simulink model "pe_pmsm_drive_code"  (R2018b)
settings: Solver=FixedStepDiscrete  StartTime=0.0  StopTime=0.5  FixedStep=2e-7  MaxStep=2.0E-6  RelTol=1e-6  AbsTol=1e-3  EnableMultiTasking=on
PreLoadFcn:
  | % Control parameters
  | Ts = 2e-6;   % Fundamental sample time
  | fsw = 2e3;   % Switching frequency (Hz)
  | fc = fsw*10; % Control loop frequency (Hz)
  | Tsc = 1/fc;  % Control loop sample time
  | 
  | % PMSM parameters
  | PM = 0.03; % Permanent magnet flux linkage
  | Ld = 2e-4;  % d-axis inductance
  | Lq = 2e-4;  % q-axis inductance
  | L0 = 2e-4;  % 0-axis inductance
  | Rs = 0.013; % Stator resistance
  | N = 6; % Number of pole pairs
  | J = 0.2; % Moment of inertia
  | 
  | % Operating and derived limits
  | Imax = 100;  % Max stator current (peak value)
  | Tmax = 1.5*N*PM*Imax; % Max lectromagnetic torque
  | fnom = 100;  % Nominal frequency (Hz)
  | rpm_nom = 60*fnom/N;      % Nominal rotor speed (rpm)
  | omegam_nom = 2*pi*fnom/N; % Nominal mechanical rotor speed
  | Pmax = omegam_nom*Tmax;     % Maximum power
values from neighbouring files (symbols this model uses):
  faero = 0.5*cd*frontarea*airdens.*speed.^2    [PMSM_code.m]
  speed = linspace(0, 60, 1000)    [PMSM_code.m]
  wheelrad = 0.3    [PMSM_code.m]
undefined symbols (not defined in the file or in its folder): DiscIntNeverNeededParam, gcbh, pe_sli_rtmsupport
libraries: nesl_utility x12, pe_lib x10, fl_lib x8, peTransforms x2, pePmsmCurrentController x1, simulink x1, peVelocityController x1
(part 1 of 2)
CloseFcn:
  | try
  |   clear Imax J L0 Ld Lq N PM Pmax Rs
  |   clear Tmax Ts Tsc fc fnom fsw
  |   clear omegam_nom rpm_nom tout
  | end
Description:
  | Three-Phase PMSM Drive
  | 
  | This example shows a Permanent Magnet Synchronous Machine
  | (PMSM) and inverter sized for use in a typical hybrid vehicle.
  | Here the inverter is connected directly to the vehicle battery, but
  | often there is also a DC-DC converter stage in between. The
  | model can be used to design the PMSM controller, selecting
  | architecture and gains to achieve desired performance. To check
  | the timing of IGBT turn-on and turn-off, the IGBT devices can be
  | directly replaced by more detailed device models from
  | Simscape(TM) Electronics(TM). For complete vehicle modeling, the
  | Simscape Electronics Servomotor block can be used to abstract
  | the PMSM, inverter and controller with an energy-based model.
  | The Gmin resistor provides a very small conductance to ground
  | that improves the numerical properties of the model when using
  | a variable-step solver.
  | 
  | Copyright 2014-2017 The MathWorks, Inc.
settings Model: Creator=The MathWorks, Inc.  LastModifiedBy=Giorgia
settings SolverCC: AutoScaleAbsTol=off  MaxConsecutiveMinStep=2  AlgebraicLoopSolver=LineSearch
settings DataIOCC: LimitDataPoints=on  SaveFormat=Array  ReturnWorkspaceOutputs=on
settings OptimizationCC: DefaultParameterBehavior=Inlined  UseDivisionForNetSlopeComputation=on  UseFloatMulNetSlope=on  InlineInvariantSignals=on  PassReuseOutputArgsAs=Individual arguments  ZeroExternalMemoryAtStartup=off  ZeroInternalMemoryAtStartup=off  NoFixptDivByZeroProtection=on  EfficientFloat2IntCast=on  LifeSpan=1  OptimizeBlockOrder=speed  DifferentSizesBufferReuse=on
settings DebuggingCC: UnderspecifiedInitializationDetection=Classic  MergeDetectMultiDrivingBlocksExec=none  MaxConsecutiveZCsMsg=none  ParameterTunabilityLossMsg=error  AllowSymbolicDim=off  LibraryContextMissingDiagnostic=none  SFUnexpectedBacktrackingDiag=warning  SFNoUnconditionalDefaultTransitionDiag=warning  SFExecutionAtInitializationDiag=none
settings HardwareCC: ProdBitPerPointer=32  ProdBitPerSizeT=32  ProdBitPerPtrDiffT=32  ProdLargestAtomicInteger=Long  ProdLargestAtomicFloat=Double  ProdWordSize=32  ProdLongLongMode=on  ProdHWDeviceType=ARM Compatible->ARM Cortex
settings ModelReferenceCC: PropagateSignalLabelsOutOfModel=off
settings SFSimCC: SimUseLocalCustomCode=off  MATLABDynamicMemAlloc=off
settings RTWCC: SystemTargetFile=autosar.tlc  GenCodeOnly=on  TemplateMakefile=ert_default_tmf  Description=AUTOSAR  GenerateReport=on  RTWUseLocalCustomCode=off  IncludeHyperlinkInReport=on  LaunchReport=on  GenerateTraceInfo=on  GenerateTraceReport=on  GenerateTraceReportSl=on  GenerateTraceReportSf=on  GenerateTraceReportEml=on  GenerateCodeMetricsReport=on
settings CodeAppCC: ForceParamTrailComments=on  IgnoreCustomStorageClasses=off  OperatorAnnotations=on  SimulinkDataObjDesc=on  SFDataObjDesc=on  CustomSymbolStrGlobalVar=rt$N$M  CustomSymbolStrType=$N$M  CustomSymbolStrFcn=$N$M$F  CustomSymbolStrMacro=$N$M  InsertBlockDesc=on
settings STFCustomTargetCC: MultiwordLength=256  ParMdlRefBuildCompliant=on  CompOptLevelCompliant=on  IncludeMdlTerminateFcn=off  CombineOutputUpdateFcns=on  CombineSignalStateStructs=on  SuppressErrorStatus=on  ERTCustomFileBanners=on  SupportNonFinite=off  SupportComplex=off  SupportContinuousTime=off  SupportNonInlinedSFcns=off  RemoveResetFunc=on  MATLABClassNameForMDSCustomization=Simulink.SoftwareTarget.ERTCustomization  AutosarCompliant=on  UseToolchainInfoCompliant=on  LookupTableObjectStructAxisOrder=2,1,3,4,...  LUTObjectStructOrderEvenSpacing=Size,Table,Breakpoints  SystemTargetFile=autosar.tlc
settings ERTTargetCC: ConcurrentExecutionCompliant=off  IncludeMdlTerminateFcn=off  CombineSignalStateStructs=on  SuppressErrorStatus=on  SupportNonFinite=off  SupportComplex=off  ModelStepFunctionPrototypeControlCompliant=off  CPPClassGenCompliant=off  AutosarCompliant=on  LookupTableObjectStructAxisOrder=2,1,3,4,...  LUTObjectStructOrderEvenSpacing=Size,Table,Breakpoints  InlinedParameterPlacement=NonHierarchical  ERTCustomFileTemplate=example_file_process.tlc
settings ConfigComp: CovMetricSettings=dw  CovHtmlReporting=on  CovSaveCumulativeToWorkspaceVar=on  CovSaveSingleToWorkspaceVar=on  CovShowResultsExplorer=off  CovExternalEMLEnable=off  CovSFcnEnable=off

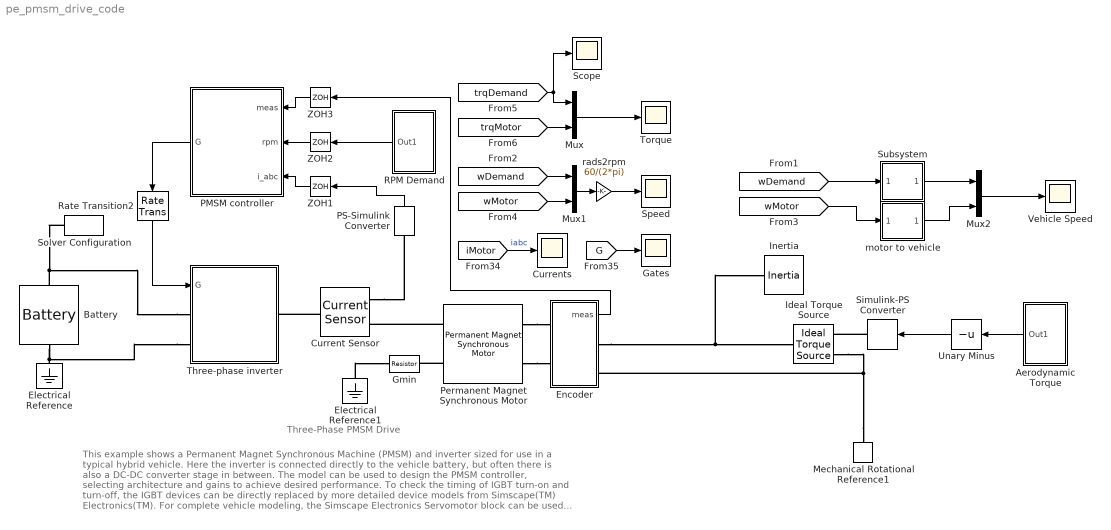
== system pe_pmsm_drive_code ==
  note: This example shows a Permanent Magnet Synchronous Machine (PMSM) and inverter sized for use in a typical hybrid vehicle.
      | Here the inverter is connected directly to the vehicle battery, but often there is also a DC-DC converter stage in between. The
      | model can be used to design the PMSM controller, selecting architecture and gains to achieve desired performance. To check
      | the timing of IGBT turn-on and turn-off, the IGBT devices can be directly replaced by more detailed device models from
      | Simscape(TM) Electronics(TM). For complete vehicle modeling, the Simscape Electronics Servomotor block can be used to
      | abstract the PMSM, inverter and controller with an energy-based model. The Gmin resistor provides a very small conductance
      | to ground that improves the numerical properties of the model when using a variable-step solver.
  note: Three-Phase PMSM Drive
  Aerodynamic Torque : Subsystem
  Battery : pe_lib/Sources/Battery  Vnom=110 V  R1=0.001 Ohm  prm_AH=1  AH=14000 hr*A  V1=470 V  AH1=5000 hr*A  prm_R2=1  R2=inf Ohm  prm_dyn=1  Rp1=0.005 Ohm  tau1=30 s  Rp2=0.005 Ohm  tau2=30 s  Rp3=0.005 Ohm  tau3=30 s  Rp4=0.005 Ohm  tau4=30 s  Rp5=0.005 Ohm  tau5=30 s  prm_fade=1  N_fade=100  AH_fade=45 hr*A  R1_fade=2.02 Ohm  V1_fade=10.35 V  i_specify=off  i_priority=None  i=0 A  i_nominal_specify=off  i_nominal_unit=A  i_nominal_value=1  v_specify=off  v_priority=None  v=0 V  v_nominal_specify=off  v_nominal_unit=V  v_nominal_value=1  charge_specify=on  charge_priority=High  charge=7000 hr*A  charge_nominal_specify=off  charge_nominal_unit=hr*A  charge_nominal_value=1  num_cycles_specify=off  num_cycles_priority=High  num_cycles=0  num_cycles_nominal_specify=off  num_cycles_nominal_unit=1  num_cycles_nominal_value=1  thermal_mass=30000 J/K  Tmeas=298.15 K  Vnom_T2=12 V  R1_T2=2.2 Ohm  V1_T2=11.4 V  R2_T2=2200 Ohm  Rp1_T2=0.005 Ohm  tau1_T2=30 s  Rp2_T2=0.005 Ohm  tau2_T2=30 s  Rp3_T2=0.005 Ohm  tau3_T2=30 s  Rp4_T2=0.005 Ohm  tau4_T2=30 s  Rp5_T2=0.005 Ohm  tau5_T2=30 s  Tmeas2=273.15 K  temperature_specify=off  temperature_priority=High  temperature=298.15 K  temperature_nominal_specify=off  temperature_nominal_unit=K  temperature_nominal_value=1
      settings: SourceProductName=Simscape Electrical  SourceProductBaseCode=PS
  Current Sensor : pe_lib/Sensors/Current Sensor
      settings: SourceProductName=Simscape Electrical  SourceProductBaseCode=PS
  Currents : Scope
  Electrical Reference : fl_lib/Electrical/Electrical Elements/Electrical Reference
      settings: SourceProductName=Foundation Library
  Electrical Reference1 : fl_lib/Electrical/Electrical Elements/Electrical Reference
      settings: SourceProductName=Foundation Library
  Encoder : Subsystem
  Gates : Scope
  Gmin : fl_lib/Electrical/Electrical Elements/Resistor  R=1e9 Ohm  i_specify=off  i_priority=High  i=0 A  i_nominal_specify=off  i_nominal_unit=A  i_nominal_value=1  v_specify=off  v_priority=High  v=0 V  v_nominal_specify=off  v_nominal_unit=V  v_nominal_value=1
      settings: SourceProductName=Foundation Library
  Ideal Torque Source : fl_lib/Mechanical/Mechanical Sources/Ideal Torque Source
  Inertia : fl_lib/Mechanical/Rotational Elements/Inertia  inertia=0.01 kg*m^2  w_specify=off  w_priority=High  w=0 rad/s  w_nominal_specify=off  w_nominal_unit=rad/s  w_nominal_value=1  t_specify=off  t_priority=None  t=0 N*m  t_nominal_specify=off  t_nominal_unit=N*m  t_nominal_value=1
  Mechanical Rotational Reference1 : fl_lib/Mechanical/Rotational Elements/Mechanical Rotational Reference
      settings: SourceProductName=Foundation Library
  Mux : Mux  Inputs=2
  Mux1 : Mux  Inputs=2
  Mux2 : Mux  Inputs=2
  PMSM controller : Subsystem
  PS-Simulink Converter : nesl_utility/PS-Simulink Converter  PhysicalDomain=network_engine_domain  SubClassName=ps_output  LeftPortType=input  RightPortType=output  PseudoPeriodic=off  Frequencies=[]  Unit=A  AffineConversion=off
  Permanent Magnet Synchronous Motor : pe_lib/Machines/Permanent Magnet Rotor/Permanent Magnet Synchronous Motor  nPolePairs=N  pmflux_param=1  pm_flux_linkage=PM Wb  torque_constant=0.18 N*m/A  back_emf_constant=0.18 V/(rad/s)  stator_param=1  Ld=Ld H  Lq=Lq H  L0=L0 H  Ls=0.0002 H  Lm=0.00002 H  Ms=0.00002 H  Rs=Rs Ohm  zero_sequence=pe.enum.park.zerosequence.include  J=0 kg*m^2  lam=0 N*m/(rad/s)  axes_param=1  i_d_specify=off  i_d_priority=None  i_d=0 A  i_d_nominal_specify=off  i_d_nominal_unit=A  i_d_nominal_value=1  i_q_specify=off  i_q_priority=None  i_q=0 A  i_q_nominal_specify=off  i_q_nominal_unit=A  i_q_nominal_value=1  torque_specify=off  torque_priority=None  torque=0 N*m  torque_nominal_specify=off  torque_nominal_unit=N*m  torque_nominal_value=1  angular_velocity_specify=on  angular_velocity_priority=None  angular_velocity=0 rpm  angular_velocity_nominal_specify=off  angular_velocity_nominal_unit=rpm  angular_velocity_nominal_value=1  angular_position_specify=on  angular_position_priority=High  angular_position=0 rad  angular_position_nominal_specify=off  angular_position_nominal_unit=deg  angular_position_nominal_value=1
      settings: SourceProductName=Simscape Electrical  SourceProductBaseCode=PS
  RPM Demand : Subsystem
  Rate Transition2 : RateTransition  Deterministic=off  OutPortSampleTime=Ts
  Scope : Scope
  Simulink-PS Converter : nesl_utility/Simulink-PS Converter  PhysicalDomain=network_engine_domain  SubClassName=ps_input  LeftPortType=input  RightPortType=output  PseudoPeriodic=off  Frequencies=[]  NoiseDistribution=none  NoiseParameters=[]  Unit=1  AffineConversion=off  FilteringAndDerivatives=provide  SimscapeFilterOrder=1  InputFilterTimeConstant=0.001  UdotUserProvided=0
  Solver Configuration : nesl_utility/Solver Configuration  PhysicalDomain=network_engine_domain  SubClassName=solver  LeftPortType=input  RightPortType=generic  Tones=[]  Harmonics=[]  SimulateNoise=off  Profile=off  UseLocalSampling=off  EnableSwitchedLinearOptims=on  FrequencyDomain=off  UseCCode=off  RelTol=0.001  AbsTol=1e-06  MinStep=1e-09  ToWorkspace=off  RevertToSquareIcSolve=off  NumHomotopyIterations=100  PhasorMode=off  PhasorModeNumHarmonics=1  DoDC=off  ResidualTolerance=1e-9  UseLocalSolver=on  LocalSolverChoice=NE_BACKWARD_EULER_ADVANCER  LocalSolverSampleTime=Ts  DoFixedCost=on  MaxNonlinIter=4  MaxModeIter=2  LinearAlgebra=Sparse  EquationFormulation=NE_TIME_EF  DelaysMemoryBudget=1024  AutomaticFiltering=on  FilteringTimeConstant=0.001  PartitionStorageMethod=AS_NEEDED  PartitionMemoryBudget=1024
  Speed : Scope
  Subsystem : Subsystem
  Three-phase inverter : Subsystem
  Torque : Scope
  Unary Minus : UnaryMinus
  "Vehicle Speed " : Scope
  ZOH1 : ZeroOrderHold  SampleTime=Tsc
  ZOH2 : ZeroOrderHold  SampleTime=Tsc
  ZOH3 : ZeroOrderHold  SampleTime=Tsc
  "motor to vehicle " : Subsystem
  rads2rpm : Gain  Gain=60/(2*pi)
  wires:
  PS-Simulink Converter/1 -> ZOH1/1
  Mux1/1 -> rads2rpm/1
  [iMotor] -> Currents/1  "iabc"
  [G] -> Gates/1
  [wDemand] -> Mux1/1
  Mux/1 -> Torque/1
  [trqMotor] -> Mux/2
  [trqDemand] -> Scope/1, Mux/1
  Encoder/1(meas) -> ZOH3/1
  ZOH3/1 -> PMSM controller/1(meas)
  ZOH2/1 -> PMSM controller/2(rpm)
  ZOH1/1 -> PMSM controller/3(i_abc)
  Rate Transition2/1 -> Three-phase inverter/1(G)
  [wMotor] -> Mux1/2
  rads2rpm/1 -> Speed/1
  PMSM controller/1(G) -> Rate Transition2/1
  Aerodynamic Torque/1(Out1) -> Unary Minus/1
  Unary Minus/1 -> Simulink-PS Converter/1
  Mux2/1 -> "Vehicle Speed "/1
  [wDemand] -> Subsystem/1(In1)
  Subsystem/1(Out1) -> Mux2/1
  [wMotor] -> "motor to vehicle "/1(In1)
  "motor to vehicle "/1(Out1) -> Mux2/2
  RPM Demand/1(Out1) -> ZOH2/1
  connections:
  Three-phase inverter/LConn1 -- Solver Configuration/RConn1 -- Battery/LConn1
  Permanent Magnet Synchronous Motor/RConn1 -- Encoder/LConn1
  Permanent Magnet Synchronous Motor/RConn2 -- Encoder/LConn2
  Current Sensor/LConn1 -- Three-phase inverter/RConn1
  Three-phase inverter/LConn2 -- Electrical Reference/LConn1 -- Battery/RConn1
  Permanent Magnet Synchronous Motor/LConn1 -- Current Sensor/RConn2
  Current Sensor/RConn1 -- PS-Simulink Converter/LConn1
  Permanent Magnet Synchronous Motor/LConn2 -- Gmin/RConn1
  Electrical Reference1/LConn1 -- Gmin/LConn1
  Encoder/RConn1 -- Ideal Torque Source/LConn1 -- Inertia/LConn1
  Mechanical Rotational Reference1/LConn1 -- Ideal Torque Source/RConn2 -- Encoder/RConn2
  Simulink-PS Converter/RConn1 -- Ideal Torque Source/RConn1

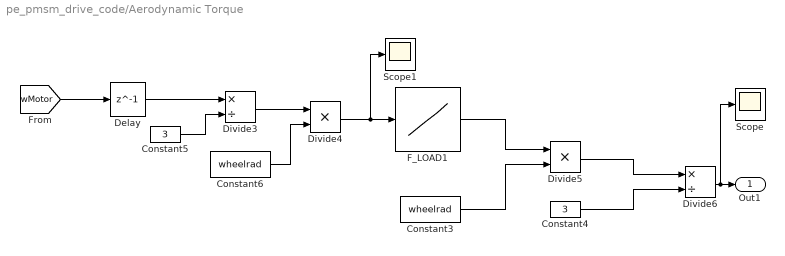
== system pe_pmsm_drive_code/Aerodynamic Torque ==
  Constant3 : Constant  Value=wheelrad
  Constant4 : Constant  Value=3
  Constant5 : Constant  Value=3
  Constant6 : Constant  Value=wheelrad
  Delay : Delay  DelayLength=1  InitialCondition=0
  Divide3 : Product  Inputs=*/
  Divide4 : Product  Inputs=**
  Divide5 : Product  Inputs=**
  Divide6 : Product  Inputs=*/
  F_LOAD1 : Lookup_n-D  NumberOfTableDimensions=1  BreakpointsForDimension1=speed  Table=faero  ExtrapMethod=Clip  RemoveProtectionInput=on  UseLastTableValue=on  InternalRulePriority=Speed  RndMeth=Simplest  InputSameDT=on
  Scope : Scope
  Scope1 : Scope
  Out1 : Outport
  wires:
  F_LOAD1/1 -> Divide5/1
  Constant3/1 -> Divide5/2
  Divide5/1 -> Divide6/1
  Constant4/1 -> Divide6/2
  Divide6/1 -> Scope/1, Out1/1
  Constant5/1 -> Divide3/2
  Delay/1 -> Divide3/1
  Divide3/1 -> Divide4/1
  Constant6/1 -> Divide4/2
  Divide4/1 -> Scope1/1, F_LOAD1/1
  [wMotor] -> Delay/1

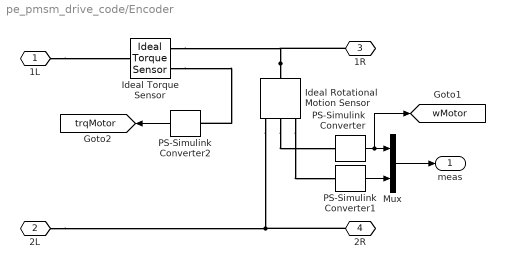
== system pe_pmsm_drive_code/Encoder ==
  Ideal Rotational Motion Sensor : fl_lib/Mechanical/Mechanical Sensors/Ideal Rotational Motion Sensor  offset=0 deg
      settings: SourceProductName=Foundation Library
  Ideal Torque Sensor : fl_lib/Mechanical/Mechanical Sensors/Ideal Torque Sensor
      settings: SourceProductName=Foundation Library
  Mux : Mux  Inputs=2
  PS-Simulink Converter : nesl_utility/PS-Simulink Converter  PhysicalDomain=network_engine_domain  SubClassName=ps_output  LeftPortType=input  RightPortType=output  PseudoPeriodic=off  Frequencies=[]  Unit=rad/s  AffineConversion=off
  PS-Simulink Converter1 : nesl_utility/PS-Simulink Converter  PhysicalDomain=network_engine_domain  SubClassName=ps_output  LeftPortType=input  RightPortType=output  PseudoPeriodic=off  Frequencies=[]  Unit=rad  AffineConversion=off
  PS-Simulink Converter2 : nesl_utility/PS-Simulink Converter  PhysicalDomain=network_engine_domain  SubClassName=ps_output  LeftPortType=input  RightPortType=output  PseudoPeriodic=off  Frequencies=[]  Unit=N*m  AffineConversion=off
  1L : PMIOPort  Side=Left
  2L : PMIOPort  Port=2  Side=Left
  1R : PMIOPort  Port=3  Side=Right
  2R : PMIOPort  Port=4  Side=Right
  meas : Outport
  tag scope: trqMotor=global, wMotor=global
  wires:
  PS-Simulink Converter2/1 -> [trqMotor]
  Mux/1 -> meas/1
  PS-Simulink Converter1/1 -> Mux/2
  PS-Simulink Converter/1 -> [wMotor], Mux/1
  connections:
  Ideal Torque Sensor/RConn2 -- PS-Simulink Converter2/LConn1
  1L/RConn1 -- Ideal Torque Sensor/LConn1
  2R/RConn1 -- 2L/RConn1 -- Ideal Rotational Motion Sensor/RConn1
  Ideal Rotational Motion Sensor/LConn1 -- 1R/RConn1 -- Ideal Torque Sensor/RConn1
  Ideal Rotational Motion Sensor/RConn2 -- PS-Simulink Converter/LConn1
  Ideal Rotational Motion Sensor/RConn3 -- PS-Simulink Converter1/LConn1

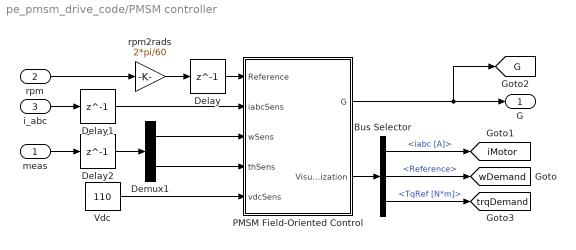
== system pe_pmsm_drive_code/PMSM controller ==
  meas : Inport
  rpm : Inport  Port=2
  i_abc : Inport  Port=3
  Bus Selector : BusSelector  OutputSignals=iabc [A],Reference,TqRef [N*m]
  Delay : Delay  DelayLength=1  InitialCondition=0
  Delay1 : Delay  DelayLength=1  InitialCondition=0
  Delay2 : Delay  DelayLength=1  InitialCondition=0
  Demux1 : Demux  Outputs=2
  PMSM Field-Oriented Control : Subsystem  AncestorBlock=pePmsmFieldOrientedControl/PMSM Field-Oriented Control  LoadFcn=pe_sli_rtmsupport( 'loadfcn', gcbh );  mask(PMSM Field-Oriented Control){CtrlMode=Velocity control, Vnom=110, Pmax=Pmax, Tmax=Tmax*1.5, p=N, Vdc_on=10, Ts=Ts, Tsc=Tsc, CtrlType=PI control, Kp_w=0.8, Ki_w=20, Kv_w=1, Kaw_w=1000, RefType=Zero d-axis control, rpmVec=[0, 3000], TqVec=[-100, 0, 100], VdcVec=[300, 350], idMatrix=zeros(2,3,2), iqMatrix=zeros(2,3,2), psim=PM, Ld=0.00024, Lq=0.00029, Rs=0.01, AxisAlignment=Q-axis, Kp_id=0.1, Ki_id=10, Kaw_id=1000, Kp_iq=0.1, Ki_iq=10, Kaw_iq=1000, AxisPrio=Q-axis, ActZC=off, ActFF=on, ParamTypeFF=Constant parameters, LdFF=Ld, LqFF=Lq, psimFF=PM, idVect=[-200, 0, 200], iqVect=[-200, 0, 200], LdMatrix=0.0002 * ones(3, 3), LqMatrix=0.0002 * ones(3, 3), psimMatrix=0.04 * ones(3, 3), CPWMMode=SPWM: sinusoidal PWM, SamplingMode=Natural, fsw=fsw}
      mask prompts: CtrlMode "Control mode:"; Vnom "Nominal dc-link voltage (V):"; Pmax "Maximum power (W):"; Tmax "Maximum torque (N*m):"; p "Number of rotor pole pairs:"; Vdc_on "Inverter dc-link voltage threshold (V):"; Ts "Fundamental sample time (s):"; Tsc "Control sample time (s):"; CtrlType "Control type:"; Kp_w "Controller proportional gain:"; Ki_w "Controller integral gain:"; Kv_w "P controller proportional gain:"; Kaw_w "Integral anti-windup gain:"; RefType "Current references:"; rpmVec "Mechanical speed vector, wMechanical (rpm):"; TqVec "Torque reference vector, TqRef (N*m):"; VdcVec "DC-link voltage vector, Vdc (V)"; idMatrix "D-axis current reference matrix, id(wMechanical,TqRef,Vdc), (A):"; iqMatrix "Q-axis current reference matrix, iq(wMechanical,TqRef,Vdc), (A):"; psim "Permanent magnet flux linkage (Wb):"; Ld "D-axis inductance (H):"; Lq "Q-axis inductance (H):"; Rs "Stator resistance (Ohm):"; AxisAlignment "Phase-a axis alignment:"; Kp_id "D-axis current proportional gain:"; Ki_id "D-axis current integral gain:"; Kaw_id "D-axis current anti-windup gain:"; Kp_iq "Q-axis current proportional gain:"; Ki_iq "Q-axis current integral gain:"; Kaw_iq "Q-axis current anti-windup gain:"; AxisPrio "Axis prioritization:"; ActZC "Enable zero cancellation"; ActFF "Enable pre-control voltage"; ParamTypeFF "Machine parameters:"; LdFF "D-axis inductance for feed-forward pre-control (H):"; LqFF "Q-axis inductance for feed-forward pre-control (H):"; psimFF "Permanent magnet flux linkage for feed-forward pre-control (Wb):"; idVect "D-axis current vector, id (A):"; iqVect "Q-axis current vector, iq (A):"; LdMatrix "Ld matrix, Ld(id,iq), (H):"; LqMatrix "Lq matrix, Lq(id,iq), (H):"; psimMatrix "Permanent magnet flux linkage matrix, PM(id,iq), (Wb):"; CPWMMode "PWM method:"; SamplingMode "Sampling mode:"; fsw "Switching frequency (Hz):"
      mask help: This block implements a PMSM field-oriented control structure.
      mask init:
      | if ParamTypeFF == 1
      |     idVect = [-200, 200];
      |     iqVect = [-200, 200];
      |     LdMatrix = LdFF*ones(2, 2);
      |     LqMatrix = LqFF*ones(2, 2);
      |     psimMatrix = psimFF*ones(2, 2);
      | end
      settings: CopyFcn=pe_sli_rtmsupport( 'copyfcn', gcbh );  DeleteFcn=pe_sli_rtmsupport( 'deletefcn', gcbh );  ModelCloseFcn=pe_sli_rtmsupport( 'modelclosefcn', gcbh );  PostSaveFcn=pe_sli_rtmsupport( 'postsavefcn', gcbh );  PreCopyFcn=pe_sli_rtmsupport( 'precopyfcn', gcbh );  OpenFcn=pe_sli_rtmsupport( 'openfcn', gcbh );  CloseFcn=pe_sli_rtmsupport( 'closefcn', gcbh );  PreDeleteFcn=pe_sli_rtmsupport( 'predeletefcn', gcbh );
      mask Help: web(nesl_help(gcbh))
      mask TypeOptions CtrlMode: Velocity control | Torque control
      mask Callback CtrlMode: pe.mask.callbackPopupPmsmFoc(gcb);
      mask TypeOptions Vnom:
      | Outer loop control/PMSM Current Reference
      | Generator/Vnom
      mask TypeOptions Pmax:
      | Outer loop control/PMSM Current Reference
      | Generator/Pmax
      mask TypeOptions Tmax:
      | Outer loop control/PMSM Current Reference
      | Generator/Tmax
      mask TypeOptions CtrlType: Outer loop control/Velocity Controller/CtrlType
      mask Callback CtrlType: pe.mask.callbackPopupPmsmFoc(gcb);
      mask TypeOptions Kp_w: Outer loop control/Velocity Controller/Kp_w
      mask TypeOptions Ki_w: Outer loop control/Velocity Controller/Ki_w
      mask TypeOptions Kv_w: Outer loop control/Velocity Controller/Kv_w
      mask TypeOptions Kaw_w: Outer loop control/Velocity Controller/Kaw_w
      mask TypeOptions RefType:
      | Outer loop control/PMSM Current Reference
      | Generator/RefType
      mask Callback RefType: pe.mask.callbackPopupPmsmFoc(gcb);
      mask TypeOptions rpmVec:
      | Outer loop control/PMSM Current Reference
      | Generator/rpmVec
      mask TypeOptions TqVec:
      | Outer loop control/PMSM Current Reference
      | Generator/TqVec
      mask TypeOptions VdcVec:
      | Outer loop control/PMSM Current Reference
      | Generator/VdcVec
      mask TypeOptions idMatrix:
      | Outer loop control/PMSM Current Reference
      | Generator/idMatrix
      mask TypeOptions iqMatrix:
      | Outer loop control/PMSM Current Reference
      | Generator/iqMatrix
      mask TypeOptions psim:
      | Outer loop control/PMSM Current Reference
      | Generator/psim
      mask TypeOptions Ld:
      | Outer loop control/PMSM Current Reference
      | Generator/Ld
      mask TypeOptions Lq:
      | Outer loop control/PMSM Current Reference
      | Generator/Lq
      mask TypeOptions Rs:
      | Outer loop control/PMSM Current Reference
      | Generator/Rs
      mask TypeOptions AxisAlignment: Inner loop control/Park Transform/AxisAlignment
      mask TypeOptions Kp_id:
      | Inner loop control/PMSM Current Controller
      | with Pre-Control/Kp_id
      mask TypeOptions Ki_id:
      | Inner loop control/PMSM Current Controller
      | with Pre-Control/Ki_id
      mask TypeOptions Kaw_id:
      | Inner loop control/PMSM Current Controller
      | with Pre-Control/Kaw_id
      mask TypeOptions Kp_iq:
      | Inner loop control/PMSM Current Controller
      | with Pre-Control/Kp_iq
      mask TypeOptions Ki_iq:
      | Inner loop control/PMSM Current Controller
      | with Pre-Control/Ki_iq
      mask TypeOptions Kaw_iq:
      | Inner loop control/PMSM Current Controller
      | with Pre-Control/Kaw_iq
      mask TypeOptions AxisPrio:
      | Inner loop control/PMSM Current Controller
      | with Pre-Control/AxisPrio
      mask TypeOptions ActZC:
      | Inner loop control/PMSM Current Controller
      | with Pre-Control/ActZC
      mask TypeOptions ActFF:
      | Inner loop control/PMSM Current Controller
      | with Pre-Control/ActFF
      mask Callback ActFF: pe.mask.callbackPopupPmsmFoc(gcb);
      mask TypeOptions ParamTypeFF: Constant parameters | Lookup table based parameters
      mask Callback ParamTypeFF: pe.mask.callbackPopupPmsmFoc(gcb);
      mask TypeOptions idVect:
      | Inner loop control/PMSM Current Controller
      | with Pre-Control/idVect
      mask TypeOptions iqVect:
      | Inner loop control/PMSM Current Controller
      | with Pre-Control/iqVect
      mask TypeOptions LdMatrix:
      | Inner loop control/PMSM Current Controller
      | with Pre-Control/LdMatrix
      mask TypeOptions LqMatrix:
      | Inner loop control/PMSM Current Controller
      | with Pre-Control/LqMatrix
      mask TypeOptions psimMatrix:
      | Inner loop control/PMSM Current Controller
      | with Pre-Control/psimMatrix
      mask TypeOptions CPWMMode:
      | PWM/PWM Generator
      | (Three-phase, Two-level)/CPWMMode
      mask TypeOptions SamplingMode:
      | PWM/PWM Generator
      | (Three-phase, Two-level)/SamplingMode
      mask DialogControl Container4 Prompt: General
      mask DialogControl Container7 Prompt: Outer Loop
      mask DialogControl Container8 Prompt: Inner Loop
      mask DialogControl Container9 Prompt: PWM
  Vdc : Constant  Value=110  SampleTime=Tsc
  rpm2rads : Gain  Gain=2*pi/60
  G : Outport
  tag scope: G=global, iMotor=global, trqDemand=global, wDemand=global
  wires:
  PMSM Field-Oriented Control/1(G) -> G/1, [G]
  Vdc/1 -> PMSM Field-Oriented Control/5(vdcSens)
  PMSM Field-Oriented Control/2(Visualization) -> Bus Selector/1
  i_abc/1 -> Delay1/1
  meas/1 -> Delay2/1
  Demux1/2 -> PMSM Field-Oriented Control/4(thSens)
  Bus Selector/1 -> [iMotor]  "<iabc [A]>"
  Bus Selector/2 -> [wDemand]  "<Reference>"
  Bus Selector/3 -> [trqDemand]  "<TqRef [N*m]>"
  rpm/1 -> rpm2rads/1
  rpm2rads/1 -> Delay/1
  Demux1/1 -> PMSM Field-Oriented Control/3(wSens)
  Delay/1 -> PMSM Field-Oriented Control/1(Reference)
  Delay1/1 -> PMSM Field-Oriented Control/2(iabcSens)
  Delay2/1 -> Demux1/1

== system pe_pmsm_drive_code/RPM Demand ==
  Constant3 : Constant  Value=wheelrad
  Constant4 : Constant  Value=3
  Divide5 : Product  Inputs=*/
  Divide6 : Product  Inputs=**
  Gain2 : Gain  Gain=30/pi
  Scope : Scope
  Scope1 : Scope
  Step : Step  Time=0.1  After=15  SampleTime=Tsc
  Out1 : Outport
  wires:
  Step/1 -> Scope/1, Divide5/1
  Constant4/1 -> Divide6/2
  Divide6/1 -> Gain2/1
  Divide5/1 -> Divide6/1
  Constant3/1 -> Divide5/2
  Gain2/1 -> Scope1/1, Out1/1

== system pe_pmsm_drive_code/Subsystem ==
  In1 : Inport
  Constant5 : Constant  Value=3
  Constant6 : Constant  Value=wheelrad
  Divide3 : Product  Inputs=*/
  Divide4 : Product  Inputs=**
  Out1 : Outport
  wires:
  Constant5/1 -> Divide3/2
  Divide3/1 -> Divide4/1
  Constant6/1 -> Divide4/2
  In1/1 -> Divide3/1
  Divide4/1 -> Out1/1

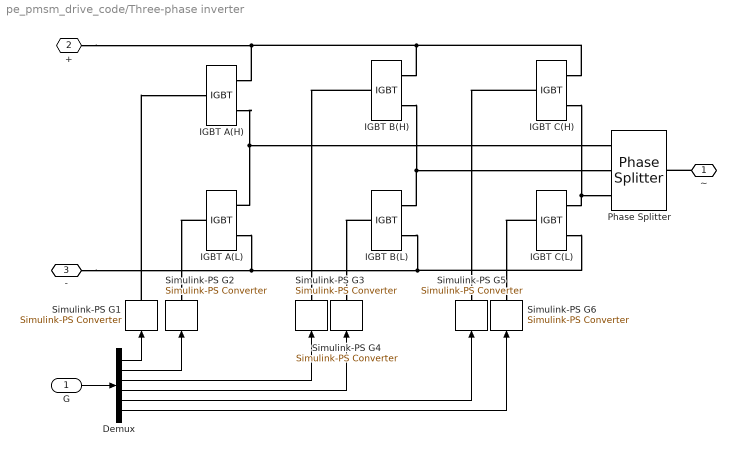
== system pe_pmsm_drive_code/Three-phase inverter ==
  G : Inport
  Demux : Demux  Outputs=6
  IGBT A(H) : pe_lib/Semiconductors/Fundamental Components/IGBT  Vf=0.8 V  Ron=0.001 Ohm  Goff=1e-5 S  Vth=0.5 V  diode_param=2  diode_Vf=0.8 V  diode_Ron=0.001 Ohm  diode_Goff=1e-5 S  diode_C=5e-8 F  diode_iRM=-235 A  diode_iF=300 A  diode_idot=-50 A/us  diode_trr_param=1  diode_trr_factor=3  diode_trr=15 us  diode_Qrr=1.5e+3 s*uA  thermal_loss_option=1  Voff=300 V  Tau=0.1 s  Tj=[ 298.15 398.15 ] K  Iout_scalar=600 A  Eon_scalar=0.02286 J  Eoff_scalar=0.01714 J  Von_scalar=2.7 V  Iout_data=[ 0 10 50 100 200 400 600 ] A  Eon_data=[ 0 2.9e-4 0.00143 0.00286 0.00571 0.01314 0.02286; 0 5.7e-4 0.00263 0.00514 0.01029 0.02057 0.03029 ] J  Eoff_data=[ 0 2.1e-4 0.00107 0.00214 0.00429 0.009859999999999999 0.01714; 0 4.3e-4 0.00197 0.00386 0.00771 0.01543 0.02271 ] J  Von_data=[ 0 1.1 1.3 1.45 1.75 2.25 2.7; 0 1 1.15 1.35 1.7 2.35 3 ] V
      settings: SourceProductName=Simscape Electrical  SourceProductBaseCode=PS
  IGBT A(L) : pe_lib/Semiconductors/Fundamental Components/IGBT  Vf=0.8 V  Ron=0.001 Ohm  Goff=1e-5 S  Vth=0.5 V  diode_param=2  diode_Vf=0.8 V  diode_Ron=0.001 Ohm  diode_Goff=1e-5 S  diode_C=5e-8 F  diode_iRM=-235 A  diode_iF=300 A  diode_idot=-50 A/us  diode_trr_param=1  diode_trr_factor=3  diode_trr=15 us  diode_Qrr=1.5e+3 s*uA  thermal_loss_option=1  Voff=300 V  Tau=0.1 s  Tj=[ 298.15 398.15 ] K  Iout_scalar=600 A  Eon_scalar=0.02286 J  Eoff_scalar=0.01714 J  Von_scalar=2.7 V  Iout_data=[ 0 10 50 100 200 400 600 ] A  Eon_data=[ 0 2.9e-4 0.00143 0.00286 0.00571 0.01314 0.02286; 0 5.7e-4 0.00263 0.00514 0.01029 0.02057 0.03029 ] J  Eoff_data=[ 0 2.1e-4 0.00107 0.00214 0.00429 0.009859999999999999 0.01714; 0 4.3e-4 0.00197 0.00386 0.00771 0.01543 0.02271 ] J  Von_data=[ 0 1.1 1.3 1.45 1.75 2.25 2.7; 0 1 1.15 1.35 1.7 2.35 3 ] V
      settings: SourceProductName=Simscape Electrical  SourceProductBaseCode=PS
  IGBT B(H) : pe_lib/Semiconductors/Fundamental Components/IGBT  Vf=0.8 V  Ron=0.001 Ohm  Goff=1e-5 S  Vth=0.5 V  diode_param=2  diode_Vf=0.8 V  diode_Ron=0.001 Ohm  diode_Goff=1e-5 S  diode_C=5e-8 F  diode_iRM=-235 A  diode_iF=300 A  diode_idot=-50 A/us  diode_trr_param=1  diode_trr_factor=3  diode_trr=15 us  diode_Qrr=1.5e+3 s*uA  thermal_loss_option=1  Voff=300 V  Tau=0.1 s  Tj=[ 298.15 398.15 ] K  Iout_scalar=600 A  Eon_scalar=0.02286 J  Eoff_scalar=0.01714 J  Von_scalar=2.7 V  Iout_data=[ 0 10 50 100 200 400 600 ] A  Eon_data=[ 0 2.9e-4 0.00143 0.00286 0.00571 0.01314 0.02286; 0 5.7e-4 0.00263 0.00514 0.01029 0.02057 0.03029 ] J  Eoff_data=[ 0 2.1e-4 0.00107 0.00214 0.00429 0.009859999999999999 0.01714; 0 4.3e-4 0.00197 0.00386 0.00771 0.01543 0.02271 ] J  Von_data=[ 0 1.1 1.3 1.45 1.75 2.25 2.7; 0 1 1.15 1.35 1.7 2.35 3 ] V
      settings: SourceProductName=Simscape Electrical  SourceProductBaseCode=PS
  IGBT B(L) : pe_lib/Semiconductors/Fundamental Components/IGBT  Vf=0.8 V  Ron=0.001 Ohm  Goff=1e-5 S  Vth=0.5 V  diode_param=2  diode_Vf=0.8 V  diode_Ron=0.001 Ohm  diode_Goff=1e-5 S  diode_C=5e-8 F  diode_iRM=-235 A  diode_iF=300 A  diode_idot=-50 A/us  diode_trr_param=1  diode_trr_factor=3  diode_trr=15 us  diode_Qrr=1.5e+3 s*uA  thermal_loss_option=1  Voff=300 V  Tau=0.1 s  Tj=[ 298.15 398.15 ] K  Iout_scalar=600 A  Eon_scalar=0.02286 J  Eoff_scalar=0.01714 J  Von_scalar=2.7 V  Iout_data=[ 0 10 50 100 200 400 600 ] A  Eon_data=[ 0 2.9e-4 0.00143 0.00286 0.00571 0.01314 0.02286; 0 5.7e-4 0.00263 0.00514 0.01029 0.02057 0.03029 ] J  Eoff_data=[ 0 2.1e-4 0.00107 0.00214 0.00429 0.009859999999999999 0.01714; 0 4.3e-4 0.00197 0.00386 0.00771 0.01543 0.02271 ] J  Von_data=[ 0 1.1 1.3 1.45 1.75 2.25 2.7; 0 1 1.15 1.35 1.7 2.35 3 ] V
      settings: SourceProductName=Simscape Electrical  SourceProductBaseCode=PS
  IGBT C(H) : pe_lib/Semiconductors/Fundamental Components/IGBT  Vf=0.8 V  Ron=0.001 Ohm  Goff=1e-5 S  Vth=0.5 V  diode_param=2  diode_Vf=0.8 V  diode_Ron=0.001 Ohm  diode_Goff=1e-5 S  diode_C=5e-8 F  diode_iRM=-235 A  diode_iF=300 A  diode_idot=-50 A/us  diode_trr_param=1  diode_trr_factor=3  diode_trr=15 us  diode_Qrr=1.5e+3 s*uA  thermal_loss_option=1  Voff=300 V  Tau=0.1 s  Tj=[ 298.15 398.15 ] K  Iout_scalar=600 A  Eon_scalar=0.02286 J  Eoff_scalar=0.01714 J  Von_scalar=2.7 V  Iout_data=[ 0 10 50 100 200 400 600 ] A  Eon_data=[ 0 2.9e-4 0.00143 0.00286 0.00571 0.01314 0.02286; 0 5.7e-4 0.00263 0.00514 0.01029 0.02057 0.03029 ] J  Eoff_data=[ 0 2.1e-4 0.00107 0.00214 0.00429 0.009859999999999999 0.01714; 0 4.3e-4 0.00197 0.00386 0.00771 0.01543 0.02271 ] J  Von_data=[ 0 1.1 1.3 1.45 1.75 2.25 2.7; 0 1 1.15 1.35 1.7 2.35 3 ] V
      settings: SourceProductName=Simscape Electrical  SourceProductBaseCode=PS
  IGBT C(L) : pe_lib/Semiconductors/Fundamental Components/IGBT  Vf=0.8 V  Ron=0.001 Ohm  Goff=1e-5 S  Vth=0.5 V  diode_param=2  diode_Vf=0.8 V  diode_Ron=0.001 Ohm  diode_Goff=1e-5 S  diode_C=5e-8 F  diode_iRM=-235 A  diode_iF=300 A  diode_idot=-50 A/us  diode_trr_param=1  diode_trr_factor=3  diode_trr=15 us  diode_Qrr=1.5e+3 s*uA  thermal_loss_option=1  Voff=300 V  Tau=0.1 s  Tj=[ 298.15 398.15 ] K  Iout_scalar=600 A  Eon_scalar=0.02286 J  Eoff_scalar=0.01714 J  Von_scalar=2.7 V  Iout_data=[ 0 10 50 100 200 400 600 ] A  Eon_data=[ 0 2.9e-4 0.00143 0.00286 0.00571 0.01314 0.02286; 0 5.7e-4 0.00263 0.00514 0.01029 0.02057 0.03029 ] J  Eoff_data=[ 0 2.1e-4 0.00107 0.00214 0.00429 0.009859999999999999 0.01714; 0 4.3e-4 0.00197 0.00386 0.00771 0.01543 0.02271 ] J  Von_data=[ 0 1.1 1.3 1.45 1.75 2.25 2.7; 0 1 1.15 1.35 1.7 2.35 3 ] V
      settings: SourceProductName=Simscape Electrical  SourceProductBaseCode=PS
  Phase Splitter : pe_lib/Connections/Phase Splitter
      settings: SourceProductName=Simscape Electrical  SourceProductBaseCode=PS
  Simulink-PS G{1..6} (6 alike) : nesl_utility/Simulink-PS Converter  PhysicalDomain=network_engine_domain  SubClassName=ps_input  LeftPortType=input  RightPortType=output  PseudoPeriodic=off  Frequencies=[]  NoiseDistribution=none  NoiseParameters=[]  Unit=1  AffineConversion=off  FilteringAndDerivatives=zero  SimscapeFilterOrder=1  InputFilterTimeConstant=1e-6  UdotUserProvided=0
  ~ : PMIOPort  Tag=PMCPort  Side=Right
  + : PMIOPort  Tag=PMCPort  Port=2  Side=Left
  - : PMIOPort  Tag=PMCPort  Port=3  Side=Left
  wires:
  Demux/6 -> Simulink-PS G6/1
  Demux/5 -> Simulink-PS G5/1
  Demux/4 -> Simulink-PS G4/1
  Demux/3 -> Simulink-PS G3/1
  Demux/2 -> Simulink-PS G2/1
  G/1 -> Demux/1
  Demux/1 -> Simulink-PS G1/1
  connections:
  IGBT C(L)/LConn1 -- Simulink-PS G6/RConn1
  IGBT C(H)/LConn1 -- Simulink-PS G5/RConn1
  IGBT B(L)/LConn1 -- Simulink-PS G4/RConn1
  IGBT B(H)/LConn1 -- Simulink-PS G3/RConn1
  IGBT A(L)/LConn1 -- Simulink-PS G2/RConn1
  -/RConn1 -- IGBT A(L)/RConn2 -- IGBT C(L)/RConn2 -- IGBT B(L)/RConn2
  IGBT A(H)/RConn2 -- IGBT A(L)/RConn1 -- Phase Splitter/RConn1
  IGBT B(L)/RConn1 -- IGBT B(H)/RConn2 -- Phase Splitter/RConn2
  IGBT C(L)/RConn1 -- IGBT C(H)/RConn2 -- Phase Splitter/RConn3
  +/RConn1 -- IGBT A(H)/RConn1 -- IGBT C(H)/RConn1 -- IGBT B(H)/RConn1
  ~/RConn1 -- Phase Splitter/LConn1
  Simulink-PS G1/RConn1 -- IGBT A(H)/LConn1

== system pe_pmsm_drive_code/motor to vehicle  ==
  In1 : Inport
  Constant5 : Constant  Value=3
  Constant6 : Constant  Value=wheelrad
  Divide3 : Product  Inputs=*/
  Divide4 : Product  Inputs=**
  Out1 : Outport
  wires:
  Constant5/1 -> Divide3/2
  Divide3/1 -> Divide4/1
  Constant6/1 -> Divide4/2
  In1/1 -> Divide3/1
  Divide4/1 -> Out1/1

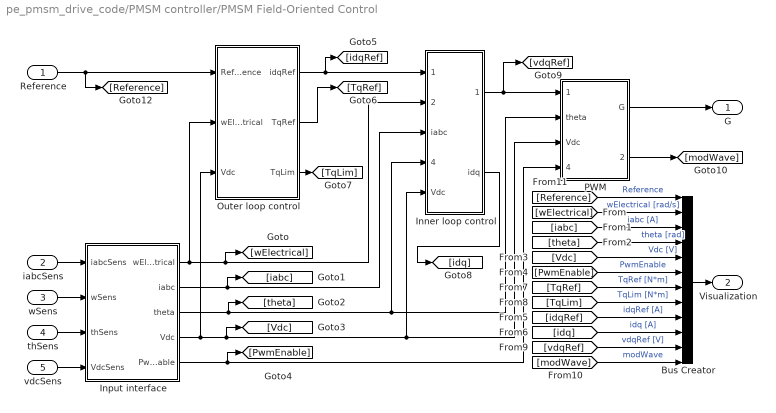
== system pe_pmsm_drive_code/PMSM controller/PMSM Field-Oriented Control ==
  Reference : Inport  SampleTime=Tsc
  iabcSens : Inport  Port=2  SampleTime=Tsc
  wSens : Inport  Port=3  SampleTime=Tsc
  thSens : Inport  Port=4  SampleTime=Tsc
  vdcSens : Inport  Port=5  SampleTime=Tsc
  Bus Creator : BusCreator  Inputs=12
  Inner loop control : Subsystem
  Input interface : Subsystem
  Outer loop control : Subsystem
  PWM : Subsystem
  G : Outport
  Visualization : Outport  Port=2
  wires:
  [modWave] -> Bus Creator/12  "modWave"
  [vdqRef] -> Bus Creator/11  "vdqRef [V]"
  [idq] -> Bus Creator/10  "idq [A]"
  [idqRef] -> Bus Creator/9  "idqRef [A]"
  [TqLim] -> Bus Creator/8  "TqLim [N*m]"
  [TqRef] -> Bus Creator/7  "TqRef [N*m]"
  [PwmEnable] -> Bus Creator/6  "PwmEnable"
  [Vdc] -> Bus Creator/5  "Vdc [V]"
  [theta] -> Bus Creator/4  "theta [rad]"
  [iabc] -> Bus Creator/3  "iabc [A]"
  [wElectrical] -> Bus Creator/2  "wElectrical [rad/s]"
  [Reference] -> Bus Creator/1  "Reference"
  PWM/2(ModWave) -> [modWave]
  Inner loop control/2(idq) -> [idq]
  Outer loop control/3(TqLim) -> [TqLim]
  Outer loop control/2(TqRef) -> [TqRef]
  Bus Creator/1 -> Visualization/1
  PWM/1(G) -> G/1
  Input interface/5(PwmEnable) -> PWM/4(PwmEnable), [PwmEnable]
  Inner loop control/1(vdqRef) -> PWM/1(vdqRef), [vdqRef]
  Input interface/1(wElectrical) -> Outer loop control/2(wElectrical), Inner loop control/2(wElectrical), [wElectrical]
  Input interface/4(Vdc) -> Outer loop control/3(Vdc), Inner loop control/5(Vdc), PWM/3(Vdc), [Vdc]
  Reference/1 -> Outer loop control/1(Reference), [Reference]
  vdcSens/1 -> Input interface/4(VdcSens)
  thSens/1 -> Input interface/3(thSens)
  wSens/1 -> Input interface/2(wSens)
  iabcSens/1 -> Input interface/1(iabcSens)
  Outer loop control/1(idqRef) -> Inner loop control/1(idq_ref), [idqRef]
  Input interface/3(theta) -> Inner loop control/4(theta), PWM/2(theta), [theta]
  Input interface/2(iabc) -> Inner loop control/3(iabc), [iabc]

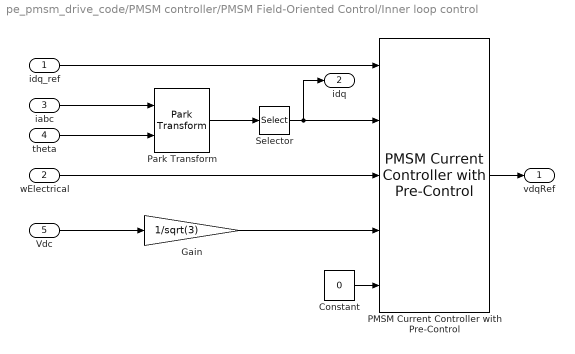
== system pe_pmsm_drive_code/PMSM controller/PMSM Field-Oriented Control/Inner loop control ==
  idq_ref : Inport
  wElectrical : Inport  Port=2
  iabc : Inport  Port=3
  theta : Inport  Port=4
  Vdc : Inport  Port=5
  Constant : Constant  Value=0  SampleTime=-1
  Gain : Gain  Gain=1/sqrt(3)
  PMSM Current Controller with Pre-Control : pePmsmCurrentController/PMSM Current Controller with Pre-Control  Kp_id=Kp_id  Ki_id=Ki_id  Kaw_id=Kaw_id  Kp_iq=Kp_iq  Ki_iq=Ki_iq  Kaw_iq=Kaw_iq  Ts=Tsc  Tsd=0.001  AxisPrio=Q-axis  ActZC=off  ActFF=on  idVect=idVect  iqVect=iqVect  LdMatrix=LdMatrix  LqMatrix=LqMatrix  psimMatrix=psimMatrix
  Park Transform : peTransforms/Park Transform  AxisAlignment=Q-axis  PowerInvariant=off
  Selector : Selector  InputPortWidth=3  IndexOptions=Index vector (dialog)  Indices=[1 2]  OutputSizes=1
  vdqRef : Outport
  idq : Outport  Port=2
  wires:
  PMSM Current Controller with Pre-Control/1 -> vdqRef/1
  Vdc/1 -> Gain/1
  wElectrical/1 -> PMSM Current Controller with Pre-Control/3
  theta/1 -> Park Transform/2
  iabc/1 -> Park Transform/1
  idq_ref/1 -> PMSM Current Controller with Pre-Control/1
  Park Transform/1 -> Selector/1
  Gain/1 -> PMSM Current Controller with Pre-Control/4
  Selector/1 -> idq/1, PMSM Current Controller with Pre-Control/2
  Constant/1 -> PMSM Current Controller with Pre-Control/5

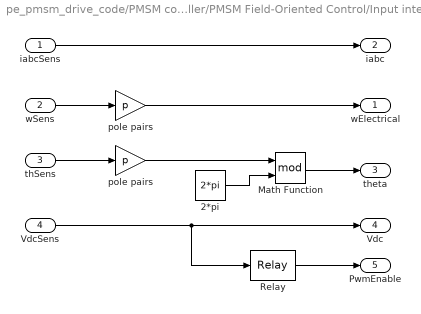
== system pe_pmsm_drive_code/PMSM controller/PMSM Field-Oriented Control/Input interface ==
  iabcSens : Inport
  wSens : Inport  Port=2
  thSens : Inport  Port=3
  VdcSens : Inport  Port=4
  2*pi : Constant  Value=2*pi  SampleTime=Tsc
  Math Function : Math  Operator=mod  SaturateOnIntegerOverflow=on
  Relay : Relay  OnSwitchValue=Vdc_on  OffSwitchValue=0.5*Vdc_on
  pole pairs : Gain  Gain=p
  "pole pairs " : Gain  Gain=p
  wElectrical : Outport
  iabc : Outport  Port=2
  theta : Outport  Port=3
  Vdc : Outport  Port=4
  PwmEnable : Outport  Port=5
  wires:
  VdcSens/1 -> Vdc/1, Relay/1
  Relay/1 -> PwmEnable/1
  Math Function/1 -> theta/1
  2*pi/1 -> Math Function/2
  "pole pairs "/1 -> Math Function/1
  iabcSens/1 -> iabc/1
  wSens/1 -> pole pairs/1
  thSens/1 -> "pole pairs "/1
  pole pairs/1 -> wElectrical/1

== system pe_pmsm_drive_code/PMSM controller/PMSM Field-Oriented Control/Outer loop control ==
  Reference : Inport
  wElectrical : Inport  Port=2
  Vdc : Inport  Port=3
  Constant : Constant  Value=0  SampleTime=-1
  PMSM Current Reference Generator : Subsystem  AncestorBlock=pePmsmCurrentReferenceGen/PMSM Current Reference Generator  LoadFcn=pe_sli_rtmsupport( 'loadfcn', gcbh );  mask(PMSM Current Reference Generator){Vnom=Vnom, Pmax=Pmax, Tmax=Tmax, Ts=Tsc, RefType=Zero d-axis control, rpmVec=rpmVec, TqVec=TqVec, VdcVec=VdcVec, idMatrix=idMatrix, iqMatrix=iqMatrix, p=p, psim=psim, Ld=Ld, Lq=Lq, Rs=Rs, RefExpEnable=0}
      mask prompts: Vnom "Nominal dc-link voltage (V):"; Pmax "Maximum power (W):"; Tmax "Maximum torque (N*m):"; Ts "Sample time (-1 for inherited):"; RefType "Current references:"; rpmVec "Mechanical speed vector, wMechanical (rpm):"; TqVec "Torque reference vector, TqRef (N*m):"; VdcVec "DC-link voltage vector, Vdc (V)"; idMatrix "D-axis current reference matrix, id(wMechanical,TqRef,Vdc), (A):"; iqMatrix "Q-axis current reference matrix, iq(wMechanical,TqRef,Vdc), (A):"; p "Number of rotor pole pairs:"; psim "Permanent magnet flux linkage (Wb):"; Ld "D-axis inductance (H):"; Lq "Q-axis inductance (H):"; Rs "Stator resistance (Ohm):"; RefExpEnable "Export current references:"
      mask help: This block implements a current reference generator for PMSM current control in the rotor d-q reference frame.
      mask init:
      | if Vnom <= 0            
      |     error(message('physmod:simscape:compiler:patterns:checks:GreaterThanZero','Nominal dc-link voltage'));            
      | end
      | 
      | if Pmax <= 0            
      |     error(message('physmod:simscape:compiler:patterns:checks:GreaterThanZero','Maximum power'));            
      | end
      | 
      | if Tmax <= 0            
      |     error(message('physmod:simscape:compiler:patterns:checks:GreaterThanZero','Maximum torque'));            
      | end
      | 
      | switch RefType
      |     case 'Zero d-axis control'
      |         EnableZDAC = 1;
      |         
      |         rpmVec = [0, 3000];
      |         TqVec  = [-100, 0, 100];
      |         VdcVec = [300, 350];
      |         idMatrix = zeros(2,3,2);
      |         iqMatrix = zeros(2,3,2);
      |     case 'Lookup-table based'
      |         EnableZDAC = 0;
      | 
      |         if length(rpmVec) < 2            
      |             error(message('physmod:simscape:compiler:patterns:checks:LengthGreaterThanOrEqual','Mechanical speed vector', '2'));            
      |         end
      |         if ~all(diff(rpmVec) > 0)            
      |             error(message('physmod:simscape:compiler:patterns:checks:StrictlyAscendingVec','Mechanical speed vector'));            
      |         end
      |         if length(TqVec) < 2            
      |             error(message('physmod:simscape:compiler:patterns:checks:LengthGreaterThanOrEqual','Torque reference vector', '2'));            
      |         end
      |         if ~all(diff(TqVec) > 0)            
      |             error(message('physmod:simscape:compiler:patterns:checks:StrictlyAscendingVec','Torque reference vector'));            
      |         end
      |         if length(VdcVec) < 2            
      |             error(message('physmod:simscape:compiler:patterns:checks:LengthGreaterThanOrEqual','DC-link voltage vector', '2'));            
      |         end
      |         if ~all(diff(VdcVec) > 0)            
      |             error(message('physmod:simscape:compiler:patterns:checks:StrictlyAscendingVec','DC-link voltage vector'));            
      |         end
      |         if ~all(size(idMatrix) == [length(rpmVec), length(TqVec), length(VdcVec)])            
      |             error(message('physmod:simscape:compiler:patterns:checks:Size3DEqual','D-axis current reference matrix', 'Mechanical speed vector', 'Torque reference vector', 'DC-link voltage vector'));            
      |         end
      |         if ~all(size(iqMatrix) == [length(rpmVec), length(TqVec), length(VdcVec)])            
      |             error(message('physmod:simscape:compiler:patterns:checks:Size3DEqual','Q-axis current reference matrix', 'Mechanical speed vector', 'Torque reference vector', 'DC-link voltage vector'));            
      |         end
      |         
      |     case 'Automatically generated lookup-table'
      |         EnableZDAC = 0;
      |         
      |         if Rs <= 0            
      |             error(message('physmod:simscape:compiler:patterns:checks:GreaterThanZero','Stator resistance'));            
      |         end
      |         if Ld <= 0            
      |             error(message('physmod:simscape:compiler:patterns:checks:GreaterThanZero','D-axis inductance'));            
      |         end
      |         if Lq <= 0            
      |             error(message('physmod:simscape:compiler:patterns:checks:GreaterThanZero','Q-axis inductance'));            
      |         end
      |         
      |         % Check if machine parameters were changed
      |         if exist('pmsm_data')
      |             dataUpdate = (pmsm_data.Ld   ~= Ld)   ||...
      |                          (pmsm_data.Lq   ~= Lq)   ||...
      |                          (pmsm_data.psim ~= psim) ||...
      |                          (pmsm_data.p    ~= p)    ||...
      |                          (pmsm_data.Rs   ~= Rs)   ||...
      |                          (pmsm_data.Pmax ~= Pmax) ||...
      |                          (pmsm_data.Tmax ~= Tmax);
      |         end
      |         
      |         % Check if grid points were changed
      |         if exist('grid_points')
      |             VecUpdate = max(abs(grid_points.RPM_VECT - rpmVec))~=0 ||...
      |                         max(abs(grid_points.TQ_VECT  - TqVec)) ~=0 ||...
      |                         max(abs(grid_points.VDC_VECT - VdcVec))~=0;
      |         end
      |         
      |         % Compute current references only IF 
      |         % current references do not exist OR 
      |         % machine parameters were changed OR
      |         % grid points were changed
      |         if ~exist('pmsm_ref') || dataUpdate || VecUpdate
      |             grid_points.RPM_VECT = rpmVec;
      |             grid_points.TQ_VECT  = TqVec;
      |             grid_points.VDC_VECT = VdcVec;
      |             pmsm_data.Ld    = Ld; 
      |             pmsm_data.Lq    = Lq; 
      |             pmsm_data.psim  = psim;   
      |             pmsm_data.p     = p;         
      |             pmsm_data.Rs    = Rs;   
      |             pmsm_data.Pmax  = Pmax;      
      |             pmsm_data.Tbase = Tmax;     
      |             pmsm_ref = pe.control.pmsm.getCurrentReferencesPmsm ( pmsm_data, grid_points );
      |             idMatrix = pmsm_ref.idMatrix;
      |             iqMatrix = pmsm_ref.iqMatrix;
      |         end
      | 
      |         % Export current references to base workspace
      |         if RefExpEnable==1
      |             assignin('base', 'pmsm_ref', pmsm_ref)
      |             set_param(gcb,'RefExpEnable','0');
      |         end
      | end
      settings: CopyFcn=pe_sli_rtmsupport( 'copyfcn', gcbh );  DeleteFcn=pe_sli_rtmsupport( 'deletefcn', gcbh );  ModelCloseFcn=pe_sli_rtmsupport( 'modelclosefcn', gcbh );  PostSaveFcn=pe_sli_rtmsupport( 'postsavefcn', gcbh );  PreCopyFcn=pe_sli_rtmsupport( 'precopyfcn', gcbh );  OpenFcn=pe_sli_rtmsupport( 'openfcn', gcbh );  CloseFcn=pe_sli_rtmsupport( 'closefcn', gcbh );  PreDeleteFcn=pe_sli_rtmsupport( 'predeletefcn', gcbh );
      mask Help: web(nesl_help(gcbh))
      mask TypeOptions RefType: Zero d-axis control | Lookup-table based | Automatically generated lookup-table
      mask Callback RefType:
      | % Callback function to set the parameters visibility
      | pe.mask.callbackPopupRefGenPmsm(gcb);
      mask DialogControl Container2 Prompt: General Parameters
      mask DialogControl Container3 Prompt: Reference Generation Strategy
      mask DialogControl RefExp Prompt: Export current references to base workspace
      mask DialogControl RefExp Callback:
      | % Enable export of current references
      | set_param(gcb,'RefExpEnable','1');
  Tq Selector : Subsystem
  Velocity Controller : peVelocityController/Velocity Controller  CtrlType=PI control  Kp_w=Kp_w  Ki_w=Ki_w  Kv_w=Kv_w  Kaw_w=Kaw_w  Ts=Tsc  Tsd=0.001  ActZC=off
  elec->mech : Gain  Gain=1/p
  idqRef : Outport
  TqRef : Outport  Port=2
  TqLim : Outport  Port=3
  wires:
  Velocity Controller/1 -> Tq Selector/2(TqRefUnsat)
  Tq Selector/1(TqRef) -> PMSM Current Reference Generator/1(TqRef)
  Constant/1 -> Velocity Controller/4
  elec->mech/1 -> Velocity Controller/2, PMSM Current Reference Generator/2(wMechanical)
  PMSM Current Reference Generator/3(TqLim) -> TqLim/1
  PMSM Current Reference Generator/2(TqRefSat) -> TqRef/1, Velocity Controller/3
  PMSM Current Reference Generator/1(idqRef) -> idqRef/1
  Vdc/1 -> PMSM Current Reference Generator/3(Vdc)
  wElectrical/1 -> elec->mech/1
  Reference/1 -> Tq Selector/1(Reference), Velocity Controller/1
